simulink model "sim_21uec072"  (R2022b)
settings: Solver=VariableStepAuto  StartTime=0.0  StopTime=0  RelTol=1e-3
settings Model: Creator=DSP-35  LastModifiedBy=DSP-35

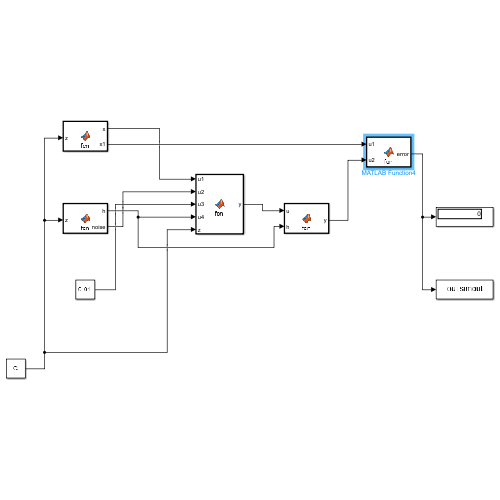
[thumbnail: Simulink's stored preview of the top-level diagram]
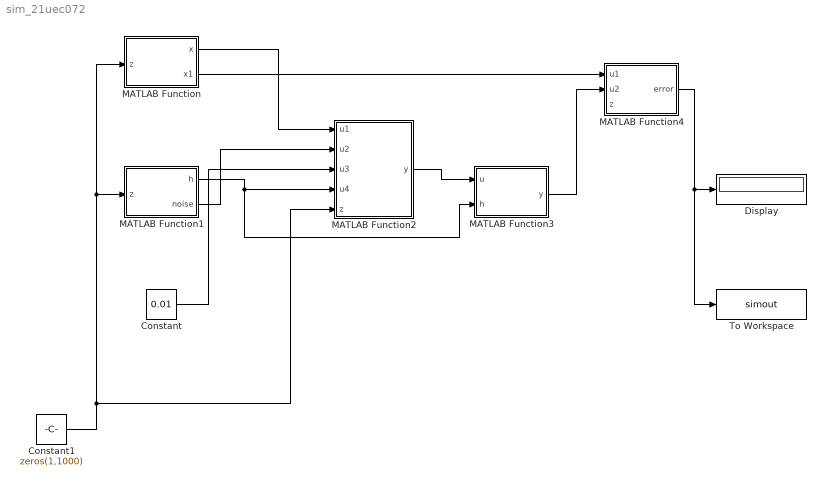
== system sim_21uec072 ==
  Constant : Constant  Value=0.01
  Constant1 : Constant  Value=zeros(1,1000)
  Display : Display
  MATLAB Function : MATLAB Function  TreatAsAtomicUnit=on
  MATLAB Function1 : MATLAB Function  TreatAsAtomicUnit=on
  MATLAB Function2 : MATLAB Function  TreatAsAtomicUnit=on
  MATLAB Function3 : MATLAB Function  TreatAsAtomicUnit=on
  MATLAB Function4 : MATLAB Function  TreatAsAtomicUnit=on
  To Workspace : ToWorkspace  VariableName=simout  SampleTime=-1
      settings: Save2DSignal=2-D array (concatenate along first dimension)
  wires:
  MATLAB Function/1(x) -> MATLAB Function2/1(u1)
  MATLAB Function1/2(noise) -> MATLAB Function2/2(u2)
  Constant/1 -> MATLAB Function2/3(u3)
  MATLAB Function4/1(error) -> To Workspace/1, Display/1
  MATLAB Function2/1(y) -> MATLAB Function3/1(u)
  MATLAB Function3/1(y) -> MATLAB Function4/2(u2)
  MATLAB Function/2(x1) -> MATLAB Function4/1(u1)
  MATLAB Function1/1(h) -> MATLAB Function3/2(h), MATLAB Function2/4(u4)
  Constant1/1 -> MATLAB Function2/5(z), MATLAB Function1/1(z), MATLAB Function/1(z)

== matlab function sim_21uec072/MATLAB Function1 ==
  data: h output; noise output; z input
function [h,noise] = fcn(z)

N = length(z);

h = (1/sqrt(2)).*complex(randn(1,N),randn(1,N));
noise = complex(randn(1,N),randn(1,N));

== matlab function sim_21uec072/MATLAB Function ==
  data: x output; x1 output; z input
function [x,x1] = fcn(z)

N = length(z);
x1 = randi(2,1,N) - 1;
x = 2*(x1) - 1;

== matlab function sim_21uec072/MATLAB Function2 ==
  data: u1 input; y output; u2 input; u3 input; u4 input; z input
function y = fcn(u1,u2,u3,u4,z)

N = length(z);
y = u1.*u4 + u2.*u3;

== matlab function sim_21uec072/MATLAB Function3 ==
  data: u input; y output; h input
function y = fcn(u,h)

y = (u./h) > 0;

== matlab function sim_21uec072/MATLAB Function4 ==
  data: u1 input; error output; u2 input; z input
function error = fcn(u1,u2,z)

N = length(z);
error = sum(abs(u1 - u2).^2)/N;
